simulink model "DQN_ABC_Test"  (R2023b)
settings: Solver=ode23tb  StartTime=0.0  StopTime=0.1  FixedStep=Ts  RelTol=1e-3
values from neighbouring files (symbols this model uses):
  Carm = 3.76    [DQn_ABC_Test_calc.m]
  L = Ld + Lm    [DQn_ABC_Test_calc.m]
  La = 1e-3    (= 0.001)    [DQn_ABC_Test_calc.m]
  Lb = 2*La    (= 0.002)    [DQn_ABC_Test_calc.m]
  Lc = 0.5*La    (= 0.0005)    [DQn_ABC_Test_calc.m]
  N = 1    [DQn_ABC_Test_calc.m]
  R = Rd + Rm    [DQn_ABC_Test_calc.m]
  Ra = 1.64    [DQn_ABC_Test_calc.m]
  Rb = 1.4*Ra    (= 2.296)    [DQn_ABC_Test_calc.m]
  Rc = 2.8*Ra    (= 4.592)    [DQn_ABC_Test_calc.m]
  Ta_dqn = oDP.Ta_dqn    [DQn_ABC_Test_calc.m]
  Ts = 50e-6    (= 5e-05)    [DQn_ABC_Test_calc.m]
  Ts_dqn = Ts    (= 5e-05)    [DQn_ABC_Test_calc.m]
  Ts_emt = Ts    (= 5e-05)    [DQn_ABC_Test_calc.m]
  Ws = 2*pi*f    (= 314.159265359)    [DQn_ABC_Test_calc.m]
undefined symbols (not defined in the file or in its folder): DiscIntNeverNeededParam, i, Xdcpnz, Xdcpnz_c, Xpnz, Ydcpnz, Ydcpnz_c, Ypnz
libraries: DQN_Lib x81, spsCurrentMeasurementLib x9, spsControlledVoltageSourceLib x9, spsSeriesRLCBranchLib x6, spsGroundLib x6, simulink x3, spsMutualInductanceLib x1, spspowerguiLib x1
(part 1 of 6)
settings Model: Creator=rober  LastModifiedBy=rober
settings SolverCC: ZeroCrossControl=DisableAll  DecoupledContinuousIntegration=on
settings DebuggingCC: UnconnectedInputMsg=warning  UnconnectedOutputMsg=warning  UnconnectedLineMsg=warning
settings ModelReferenceCC: EnableRefExpFcnMdlSchedulingChecks=on
settings RTWCC: DLArmComputeVersion=19.05

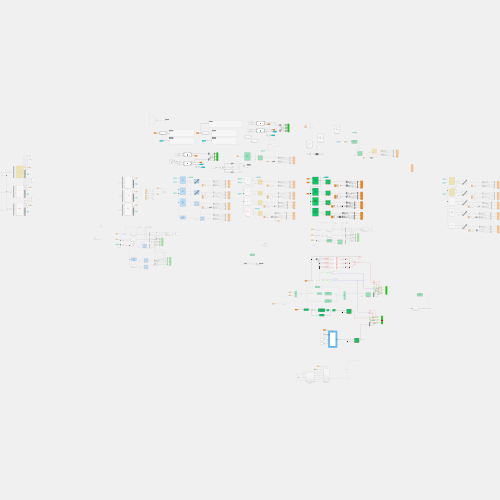
[thumbnail: Simulink's stored preview of the top-level diagram]
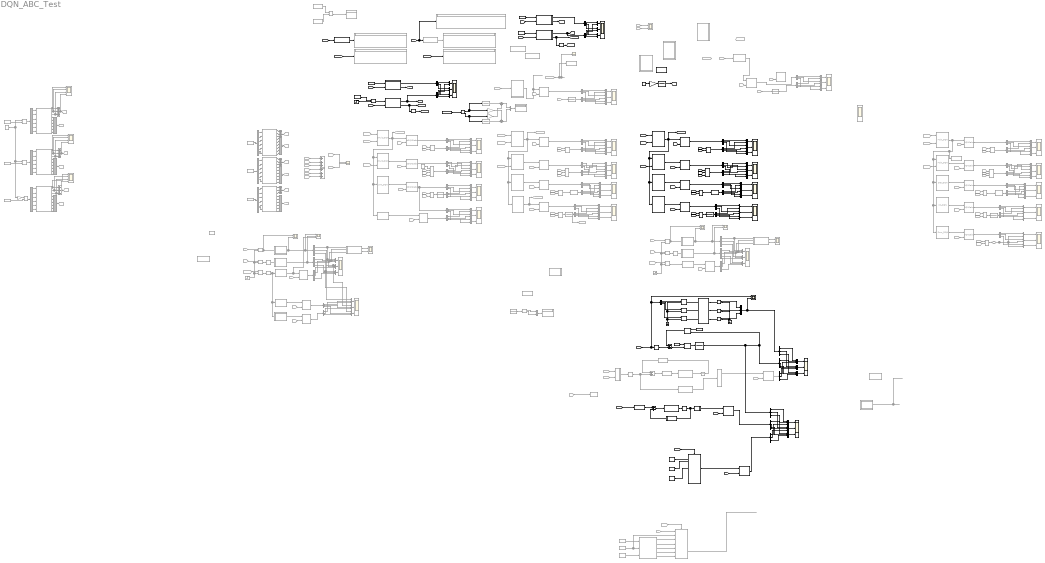
== system DQN_ABC_Test ==
  ABC : Subsystem  Commented=on
  ABC1 : Subsystem  Commented=on
  ABC2 : Subsystem  Commented=on
  Add{1..4,20..21,26..27} (8 alike) : Sum  Commented=on  Inputs=+++
  Add13 : Sum  Inputs=-+
  Add16 : Sum  Commented=on  Inputs=-+
  Add5 : Sum
  Complex to Real-Imag : ComplexToRealImag
  Complex to Real-Imag1 : ComplexToRealImag  Commented=on
  Constant : Constant  Commented=on
  Constant1 : Constant  Value=Xdcpnz
  Constant10 : Constant  Commented=on  Value=Xpnz(:,3)
  Constant11 : Constant  Value=Xdcpnz_c(1,2)
  Constant12 : Constant  Value=R
  Constant13 : Constant  Value=Xdcpnz_c
  Constant14 : Constant  Value=inv(L)
  Constant15 : Constant
  Constant16 : Constant  Value=-R/(L)
  Constant17 : Constant  Commented=on  Value=Ypnz(:,2)
  Constant18 : Constant  Commented=on  Value=Ypnz(:,3)
  Constant19 : Constant  Value=eye(3)/L
  Constant2 : Constant  Value=Ydcpnz
  Constant20 : Constant  Value=eye(3)
  Constant21 : Constant  Commented=on  Value=-R/(L)
  Constant22 : Constant  Commented=on  Value=eye(3)/L
  Constant23 : Constant  Commented=on  Value=eye(3)
  Constant3 : Constant  Commented=on
  Constant4 : Constant  Commented=on  Value=Ypnz(:,1)
  Constant5 : Constant  Value=Ydcpnz_c
  Constant6 : Constant  Commented=on  Value=Xpnz(:,1)
  Constant7 : Constant  Commented=on  Value=[1 -2 3]
  Constant8 : Constant  Commented=on  Value=[1.4 -2.8 -0.45]
  Constant9 : Constant  Commented=on  Value=Xpnz(:,2)
  Current Measurement3 : spsCurrentMeasurementLib/Current Measurement  PhasorSimulation=off  OutputType=Complex  PSBequivalent=0
  Current Measurement4 : spsCurrentMeasurementLib/Current Measurement  PhasorSimulation=off  OutputType=Complex  PSBequivalent=0
  Current Measurement5 : spsCurrentMeasurementLib/Current Measurement  PhasorSimulation=off  OutputType=Complex  PSBequivalent=0
  DQN : Subsystem  Commented=on
  DQN2abc{5,7..9} (4 alike) : DQN_Lib/DQN2abc  Commented=on  HrmOrd=2*N
  DQN2abc6 : DQN_Lib/DQN2abc  Commented=on  HrmOrd=4*N
  DQn->ABC1 : DQN_Lib/DQn->ABC19  Commented=on  N=4*N
  DQn->ABC10 : DQN_Lib/DQn->ABC19  Commented=on  N=N
  DQn->ABC{4,9,11,13} (4 alike) : DQN_Lib/DQn->ABC6  Commented=on  N=N
  DQn->ABC12 : DQN_Lib/DQn->ABC6  N=N
  DQn->ABC14 : DQN_Lib/DQn->ABC6  N=N
  DQn->ABC19 : DQN_Lib/DQn->ABC19  Commented=on  N=2*N
  DQn->ABC2 : DQN_Lib/DQn->ABC19  Commented=on  N=2*N
  DQn->ABC3 : DQN_Lib/DQn->ABC19  Commented=on  N=2*N
  DQn->ABC5 : DQN_Lib/DQn->ABC6  N=4*N
  DQn->ABC6 : DQN_Lib/DQn->ABC6  N=2*N
  DQn->ABC7 : DQN_Lib/DQn->ABC6  N=2*N
  DQn->ABC8 : DQN_Lib/DQn->ABC6  N=2*N
  Demux{,5,14..15,26..27} (6 alike) : Demux  Commented=on  Outputs=[1, 1, 1, 1, 1, 1]
  Demux{1..4,6..11,13,16..25,28..30,32..33,44..54} (37 alike) : Demux  Commented=on  Outputs=3
  Demux{12,31,34..43,55..61} (19 alike) : Demux  Outputs=3
  Demux_DQNc_Mat : DQN_Lib/Demux_DQNc_Mat  Commented=on  nrOut=2
  Der_DQN1 : DQN_Lib/Der_DQN  Commented=on  HrmOrd=2*N  FreqRad=2*pi*50  Ts=Ts_dqn  EMT=on  sw_soft=off  chkHrmLst=off  HrmLst=[7 14]
  Der_DQN_Mat : DQN_Lib/Der_DQN_Mat  Commented=on  N=2*N  w=Ws  Ts=Ts  EMT=on  sw_soft=on
  Der_DQNc_Mat : MATLAB Function  Commented=on  TreatAsAtomicUnit=on  mask{Ts=Ts, N=N, w=Ws, EMT=off, Init=zeros(3,1)}
      mask prompts: Ts "Time step (s):"; N "Harmonic order:"; w "Angular frequency [1/rad]:"; Init "Initial conditions:"
  Der_DQNc_Mat1 : DQN_Lib/Der_DQNc_Mat  Ts=Ts  N=2*N  w=Ws  EMT=on  sw_soft=on
  Discrete Derivative : simulink/Discrete/Discrete Derivative  Commented=on  gainval=1.0  ICPrevScaledInput=0.0  OutMin=[]  OutMax=[]  OutDataType=fixdt(1, 16)  OutScaling=2^-10  DoSatur=off
  Discrete Derivative1 : simulink/Discrete/Discrete Derivative  Commented=on  gainval=1.0  ICPrevScaledInput=0.0  OutMin=[]  OutMax=[]  OutDataType=fixdt(1, 16)  OutScaling=2^-10  DoSatur=off
  Discrete Derivative2 : simulink/Discrete/Discrete Derivative  gainval=1.0  ICPrevScaledInput=0.0  OutMin=[]  OutMax=[]  OutDataType=fixdt(1, 16)  OutScaling=2^-10  DoSatur=off
  Discrete-Time Integrator{,1,3,5..7,9} (7 alike) : DiscreteIntegrator  Commented=on  IntegratorMethod=Integration: Trapezoidal  SampleTime=Ts  ICPrevOutput=DiscIntNeverNeededParam  ICPrevScaledInput=DiscIntNeverNeededParam
  Discrete-Time Integrator15 : DiscreteIntegrator  IntegratorMethod=Integration: Trapezoidal  gainval=1  SampleTime=Ts_dqn  UpperSaturationLimit=5000  LowerSaturationLimit=500  ICPrevOutput=DiscIntNeverNeededParam  ICPrevScaledInput=DiscIntNeverNeededParam
  Discrete-Time Integrator2 : DiscreteIntegrator  IntegratorMethod=Integration: Trapezoidal  SampleTime=Ts  ICPrevOutput=DiscIntNeverNeededParam  ICPrevScaledInput=DiscIntNeverNeededParam
  Discrete-Time Integrator4 : DiscreteIntegrator  IntegratorMethod=Integration: Trapezoidal  SampleTime=Ts  ICPrevOutput=DiscIntNeverNeededParam  ICPrevScaledInput=DiscIntNeverNeededParam
  Discrete-Time Integrator8 : DiscreteIntegrator  Commented=on  IntegratorMethod=Integration: Trapezoidal  InitialCondition=[0.8 0.6 -0.33]  SampleTime=Ts  ICPrevOutput=DiscIntNeverNeededParam  ICPrevScaledInput=DiscIntNeverNeededParam
  Discretize BE or Tustin1 : Subsystem  Commented=on
  Display{,1,4..9} (8 alike) : Display  Commented=on
      Display settings: Decimation=1000
      Display1 settings: Decimation=1000
      Display5 settings: Decimation=1000
      Display6 settings: Decimation=1000
      Display7 settings: Decimation=1000
      Display8 settings: Decimation=1000
      Display9 settings: Decimation=1000
  EMT : Subsystem  Commented=on
  EMT1 : Subsystem  Commented=on
  Error calc : Subsystem  Commented=on
  Error calc1 : Subsystem  Commented=on
  From : From  Commented=on  GotoTag=X_DQN_mat
  From1 : From  Commented=on  GotoTag=X_DQN_vec
  From{8,10..11,15,20,43..44,46,48,50,52,54..55,57..59,81} (17 alike) : From  Commented=on  GotoTag=Yabc
  From{66,73,97,99..100,102} (6 alike) : From  Commented=on  GotoTag=Xpnz_c
  From{2,7,9,14,19,21..22,37..38,42,45,47,51,53,56,60,67,69,94..95,103..104} (22 alike) : From  Commented=on  GotoTag=Xabc
  From112 : From  Commented=on  GotoTag=X_DQN_vec
  From{3,6,12..13,16..18,30,35..36,39..41,64,72,78,89..90,98,252,262} (21 alike) : From  Commented=on  GotoTag=th0  TagVisibility=global
  From23 : From  Commented=on  GotoTag=Xabc1
  From24 : From  Commented=on  GotoTag=X_DQN_vec
  From26 : From  Commented=on  GotoTag=Xabc2
  From27 : From  Commented=on  GotoTag=Xabc3
  From28 : From  Commented=on  GotoTag=Yabc1
  From31 : From  Commented=on  GotoTag=Yabc2
  From32 : From  Commented=on  GotoTag=Yabc3
  From{4..5,33..34} (4 alike) : From  Commented=on  GotoTag=Y_DQN_vec
  From61 : From  Commented=on  GotoTag=Y_DQN_mat
  From62 : From  Commented=on  GotoTag=Y_DQN_mat
  From65 : From  Commented=on  GotoTag=iX_DQN_mat
  From68 : From  Commented=on  GotoTag=X_DQN_mat
  Gain : Gain  Gain=2*pi*50
  Gain1 : Gain  Commented=on  Gain=1/Ws
  Gain2 : Gain  Commented=on  Gain=1/Ws
  Gain8 : Gain  Commented=on
  Gain_DQNc_Mat : DQN_Lib/Gain_DQNc_Mat  Commented=on  Rabc=[R zeros(3,3); zeros(3,3) R]  HRM=N  chkInv=off
  Gain_DQNc_Mat1 : DQN_Lib/Gain_DQNc_Mat  Commented=on  Rabc=[inv(L) zeros(3,3); zeros(3,3) inv(L)]  HRM=N  chkInv=off
  Gain_DQNc_Mat2 : MATLAB Function  TreatAsAtomicUnit=on  SystemSampleTime=Ts  mask{Rabc=eye(3), HRM=N, chkInv=off}
      mask prompts: Rabc "Line matrix [3x3]:"; HRM "Harmonic order:"; chkInv "Invert"
  Gain_DQNc_Mat3 : MATLAB Function  Commented=on  TreatAsAtomicUnit=on  mask{Rabc=[L zeros(3,3); zeros(3,3) L], HRM=N, chkInv=on}
      mask prompts: Rabc "Line matrix [3x3]:"; HRM "Harmonic order:"; chkInv "Invert"
  Gain_DQNc_Mat4 : MATLAB Function  TreatAsAtomicUnit=on  SystemSampleTime=Ts  mask{Rabc=-R/(L), HRM=N, chkInv=off}
      mask prompts: Rabc "Line matrix [3x3]:"; HRM "Harmonic order:"; chkInv "Invert"
  Gain_DQNc_Mat5 : MATLAB Function  TreatAsAtomicUnit=on  SystemSampleTime=Ts  mask{Rabc=eye(3)/L, HRM=N, chkInv=off}
      mask prompts: Rabc "Line matrix [3x3]:"; HRM "Harmonic order:"; chkInv "Invert"
  Goto10 : Goto  Commented=on  GotoTag=Ydqn3
  Goto14 : Goto  Commented=on  GotoTag=XY_DQN_mat
  Goto16 : Goto  Commented=on  GotoTag=dXY_DQN_mat
  Goto17 : Goto  Commented=on  GotoTag=IntXYabc
  Goto18 : Goto  Commented=on  GotoTag=iX_DQN_mat
  Goto19 : Goto  Commented=on  GotoTag=Xabc2
  Goto2 : Goto  Commented=on  GotoTag=XY_DQN_vec
  Goto28 : Goto  Commented=on  GotoTag=Yabc2
  Goto3 : Goto  Commented=on  GotoTag=Xdqn1
  Goto32 : Goto  Commented=on  GotoTag=Xabc3
  Goto33 : Goto  Commented=on  GotoTag=Yabc3
  Goto34 : Goto  Commented=on  GotoTag=Xabc1
  Goto4 : Goto  Commented=on  GotoTag=Xdqn2
  Goto5 : Goto  Commented=on  GotoTag=Xdqn3
  Goto7 : Goto  Commented=on  GotoTag=Ydqn1
  Goto8 : Goto  Commented=on  GotoTag=Yabc1
  Goto9 : Goto  Commented=on  GotoTag=Ydqn2
  Ground2 : spsGroundLib/Ground  LConnTagsString=a
  Ground3 : spsGroundLib/Ground  LConnTagsString=a
  Ihistory_Flux : Subsystem  mask{A=-R/L, B=eye(3)/L, C=eye(3), D=zeros(3,3), Ws=2*pi*50, Ts=50e-6}
      mask prompts: Ws "Angular frequency (rad/s):"; Ts "Time step (s):"
      mask init:
      | I = eye(size(A,1));
      |     INVR = I/(I-A*Ts/2);
      |     Ad1 = INVR*(I+A*Ts/2);
      |     Bd1 = INVR*B;
      |     Cd1 = C*INVR*Ts;
      |     Dd1 = Cd1*B/2;
      | 
      |     a  = -0.5 + 1i*sqrt(3)/2;
      |     a2 = -0.5 - 1i*sqrt(3)/2;
      |     Sas = [1,a,a2;1,a2,a;1,1,1]/3;
      | 
      |     Ac = Sas*A/Sas;
      |     Bc = Sas*B/Sas;
      |     Cc = Sas*C/Sas;
      | 
      |     Ac = diag(diag(real(Ac)));
      |     Bc = diag(diag(real(Bc)));
      |     Cc = diag(diag(real(Cc)));
      settings: PortSchema="{\"entries\":[{\"content\":{\"sides\":[{\"content\":{},\"type\":\"ConnectorPlacement.EquallySpacedRectSide\",\"uuid\":\"e88392ce-eae4-4263-a591-d3f621c138f8\"},{\"content\":{\"connectorIds\":[\"Out1\"],\"side\":\"RIGHT\"},\"type\":\"ConnectorPlacement.EquallySpacedRectSide\",\"uuid\":\"cf9a43c2-5915-48ea-a98e-97bd8467efe9\"},{\"content\":{\"connectorIds\":[\"In1\"],\"side\":\"TOP\"},\"type\":\"ConnectorPlacement.EquallySpacedRectSide\",\"uuid\":\"6e30664c-e4b1-4c2e-802d-ada5c87750e1\"}]},\"type\":\"ConnectorPlacement.EquallySpacedConnector\",\"uuid\":\"d551c040-d9c0-4e4e-a3d2-ba73f5d429f0\"}],\"packageUris\":[\"http://schema.mathworks.com/mf0/Connector/R2020b\"],\"version\":\"1.0\"}"
  Ihistory_Flux1 : Subsystem  Commented=on
      settings: PortSchema="{\"entries\":[{\"content\":{\"sides\":[{\"content\":{\"connectorIds\":[\"In1\",\"In2\",\"In3\",\"In4\",\"In5\",\"In6\",\"In7\"]},\"type\":\"ConnectorPlacement.EquallySpacedRectSide\",\"uuid\":\"e88392ce-eae4-4263-a591-d3f621c138f8\"},{\"content\":{\"connectorIds\":[\"Out1\",\"Out2\"],\"side\":\"RIGHT\"},\"type\":\"ConnectorPlacement.EquallySpacedRectSide\",\"uuid\":\"cf9a43c2-5915-48ea-a98e-97bd8467efe9\"},{\"content\":{\"connectorIds\":[\"In8\"],\"side\":\"TOP\"},\"type\":\"ConnectorPlacement.EquallySpacedRectSide\",\"uuid\":\"6e30664c-e4b1-4c2e-802d-ada5c87750e1\"}]},\"type\":\"ConnectorPlacement.EquallySpacedConnector\",\"uuid\":\"d551c040-d9c0-4e4e-a3d2-ba73f5d429f0\"}],\"packageUris\":[\"http://schema.mathworks.com/mf0/Connector/R2020b\"],\"version\":\"1.0\"}"
  Int_DQN1 : DQN_Lib/Int_DQN  Commented=on  HrmOrd=2*N  FreqRad=2*pi*50  TimeStep=Ts_dqn  Init=0*(Ta_dqn*[0.01; -0.02; 0.03])'  EMT=on  chkHrmLst=off  HrmLst=[0 7 14]
  Int_DQN_Mat : DQN_Lib/Int_DQN_Mat  Commented=on  N=2*N  dt=Ts  w=Ws  EMT=off  InitInt=zeros(1,6)
  Int_DQN_Mat2 : MATLAB Function  Commented=on  TreatAsAtomicUnit=on  mask{N=N, dt=Ts, w=Ws, EMT=on, InitInt=zeros(1,6)}
      mask prompts: N "Order number:"; dt "Time step (s):"; w "Angular frequency (1/rad):"; InitInt "Initial conditions [1x6]:"
  Int_DQN_Mat4 : MATLAB Function  Commented=on  TreatAsAtomicUnit=on  mask{N=N, dt=Ts, w=Ws, EMT=on, InitInt=[0.8; 0.6; -0.33]}
      mask prompts: N "Order number:"; dt "Time step (s):"; w "Angular frequency (1/rad):"; InitInt "Initial conditions DC [3x1]:"
  Int_DQN_fdbk : DQN_Lib/Int_DQN_fdbk  Commented=on  HrmOrd=N  FreqRad=Ws  TimeStep=Ts_dqn  swFeed=on  R=Ra  iL=1/La
  Int_DQN_fdbk2 : Subsystem  Commented=on  mask{HrmOrd=N, FreqRad=Ws, TimeStep=Ts_dqn, swFeed=on, R=Ra, iL=1/La}
      mask prompts: HrmOrd "Harmonic order:"; FreqRad "Angular frequency (rad/s);"; TimeStep "Time step (s):"; swFeed "Enable feedback"; R "Feedback parameter (Kr):"; iL "Integrator parameter (Kl):"
      mask Callback swFeed:
      | EMT = get_param(gcb,'swFeed');
      | 
      | if(strcmp(EMT,'on'))
      |    set_param(gcb,'MaskVisibilities',{'on','on','on','on','on','on'});
      | else
      |    set_param(gcb,'MaskVisibilities',{'on','on','on','on','off','off'});
      | end
      mask Display:
      | %plot([0 1])
      | port_label('input',1,'{X}');
      | port_label('output',1,'{Z}');
      | 
      | harm = get_param(gcb, 'HrmOrd');
      | disp(['{\color{black}\bf\fontsize{12}Hi:',(harm),'}',newline,'{\color{red}\bf\fontsize{12}\{Int-fdbk\}}',newline,'{\color{black}\bf\fontsize{12}Ho:',(harm),'}',newline,'{\color{gray}\bf\fontsize{12}EMT}'], 'texmode','on');
  Int_DQNc_Mat : DQN_Lib/Int_DQNc_Mat  Commented=on  N=N  dt=Ts_dqn  w=Ws  InitInt=0*[0.8; 0.6; -0.33]  swFeed=on  R=diag([Ra,Rb,Rc])  iL=diag([inv(La),inv(La),inv(La)])
  Int_DQNc_Mat1 : DQN_Lib/Int_DQNc_Mat  N=2*N  dt=Ts  w=Ws  InitInt=0*[0.8; 0.6; -0.33]  swFeed=off  R=1  iL=1
  Int_DQNc_Mat2 : MATLAB Function  Commented=on  TreatAsAtomicUnit=on  mask{N=N, dt=Ts, w=Ws, InitInt=[0.8; 0.6; -0.33], swFeed=off, Ra=1, iL=1}
      mask prompts: N "Order number:"; dt "Time step (s):"; w "Angular frequency (1/rad):"; InitInt "Initial conditions DC [3x1]:"; swFeed "Enable feedback"; Ra "Feedback parameter (Kr):"; iL "Feedback parameter (Ki):"
  Int_DQNc_Mat3 : DQN_Lib/Int_DQNc_Mat  Commented=on  N=N  dt=Ts_dqn  w=Ws  InitInt=0*[0.8; 0.6; -0.33]  swFeed=off  R=Ra  iL=1/La
  Int_DQNc_Mat4 : MATLAB Function  TreatAsAtomicUnit=on  mask{N=N, dt=Ts_dqn, w=Ws, InitInt=zeros(3,1), swFeed=off, R=R/(L), iL=eye(size(-R/(L),1))}
      mask prompts: N "Order number:"; dt "Time step (s):"; w "Angular frequency (1/rad):"; InitInt "Initial conditions DC [3x1]:"; swFeed "Enable feedback"; R "Feedback parameter (Kr {abc}):"; iL "Feedback parameter (Ki {abc}):"
  Int_DQNc_Mat5 : DQN_Lib/Int_DQNc_Mat  Commented=on  N=N  dt=Ts_dqn  w=Ws  InitInt=zeros(3,1)  swFeed=on  R=[R zeros(3,3); zeros(3,3) R]  iL=[inv(L) zeros(3,3); zeros(3,3) inv(L)]
  Int_DQNc_Mat6 : DQN_Lib/Int_DQNc_Mat  Commented=on  N=N  dt=Ts_dqn  w=Ws  InitInt=zeros(3,1)  swFeed=off  R=1  iL=1
  MATLAB Function1 : MATLAB Function  TreatAsAtomicUnit=on  mask{chkHrmLst=off, HRM=N, HrmLst=[0 7 8]}
      mask prompts: chkHrmLst "Only specific harmonics"; HRM "Harmonic order:"; HrmLst "Harmonic list:"
  MATLAB Function2 : DQN_Lib/MATLAB Function4  Commented=on  SystemSampleTime=-1  VariantActivationTime=update diagram  AllowFlexibleInterface=on  Latency=0  AutoFrameSizeCalculation=off
  MATLAB Function3 : MATLAB Function  TreatAsAtomicUnit=on  mask{chkHrmLst=off, HRM=N, HrmLst=[0 7 8]}
      mask prompts: chkHrmLst "Only specific harmonics"; HRM "Harmonic order:"; HrmLst "Harmonic list:"
  MATLAB Function4 : MATLAB Function  TreatAsAtomicUnit=on  mask{chkHrmLst=off, HRM=N, HrmLst=[0 7 8]}
      mask prompts: chkHrmLst "Only specific harmonics"; HRM "Harmonic order:"; HrmLst "Harmonic list:"
  MATLAB Function6 : DQN_Lib/MATLAB Function4  SystemSampleTime=-1  VariantActivationTime=update diagram  AllowFlexibleInterface=on  Latency=0  AutoFrameSizeCalculation=off
  MATLAB Function7 : DQN_Lib/MATLAB Function4  Commented=on  SystemSampleTime=-1  VariantActivationTime=update diagram  AllowFlexibleInterface=on  Latency=0  AutoFrameSizeCalculation=off
  MATLAB Function8 : MATLAB Function  TreatAsAtomicUnit=on  mask{chkHrmLst=off, HRM=N, HrmLst=[0 7 8]}
      mask prompts: chkHrmLst "Only specific harmonics"; HRM "Harmonic order:"; HrmLst "Harmonic list:"
  MATLAB Function9 : DQN_Lib/MATLAB Function4  Commented=on  SystemSampleTime=-1  VariantActivationTime=update diagram  AllowFlexibleInterface=on  Latency=0  AutoFrameSizeCalculation=off
  Matrix Multiply8 : Product  Multiplication=Matrix(*)
  Matrix Multiply9 : Product  Multiplication=Matrix(*)
  Mult_DQN2 : DQN_Lib/Mult_DQN  Commented=on  HrmOrd=N  HrmDbl=on  chkHrmLst=off  HrmLstX=[0 7 8]  HrmLstY=[0 7 8]
  Mult_DQN3 : DQN_Lib/Mult_DQN  Commented=on  HrmOrd=2*N  HrmDbl=on  chkHrmLst=off  HrmLstX=[0 7 8 14 15 16]  HrmLstY=[0 7 8]
  Mult_DQN_Mat : DQN_Lib/Mult_DQN_Mat  Commented=on  N=N  HrmDbl=on
  Mult_DQN_Mat1 : DQN_Lib/Mult_DQN_Mat  Commented=on  N=2*N  HrmDbl=on
  Mult_DQN_Mat4 : MATLAB Function  Commented=on  TreatAsAtomicUnit=on  mask{N=N, HrmDbl=on}
      mask prompts: N "Harmonic order:"; HrmDbl "Double Harmonic"
  Mult_DQNc_Mat1 : DQN_Lib/Mult_DQNc_Mat  N=N  HrmDbl=on
  Mult_DQNc_Mat2 : DQN_Lib/Mult_DQNc_Mat  N=2*N  HrmDbl=on
  Mutual Inductance1 : spsMutualInductanceLib/Mutual Inductance  LConnTagsString=a|b|c  RConnTagsString=A|B|C  TypeOfMutual=Generalized mutual inductance  NumberOfWindings=3  SelfImpedance1=[1.1 1.1e-03]  SelfImpedance2=[ 1.1 1.1e-03]  ThreeWindings=on  SelfImpedance3=[ 1.1 1.1e-03]  MutualImpedance=[1.0 1.0e-03]  InductanceMatrix=L  ResistanceMatrix=R  Measurements=None
  Mux{,1..6,8..10,13..14,18..21,23..25,28..29,31,33..35,37..40,44..51,53..56,71..76} (47 alike) : Mux  Commented=on  Inputs=2
  Mux{7,11..12,52,57..70} (18 alike) : Mux  Inputs=2
  Mux{15..17,22,26,30} (6 alike) : Mux  Commented=on  Inputs=[1, 1, 1, 1, 1, 1]
  Mux{27,32,36,41..43,77..79} (9 alike) : Mux  Commented=on  Inputs=3
  Mux{80..86} (7 alike) : Mux  Inputs=3
  Mux_DQNc_Mat : Subsystem  Commented=on  mask{nrInp=2}
      mask prompts: nrInp "Number of inputs [{C}]"
      mask init:
      | %blocks = find_system(gcb,'LookUnderMasks','on','FollowLinks','on')
      | %set_param(gcb, 'MaskSelfModifiable', 'on');
      | 
      | % if(SSM == [])
      | %     Simulink.SubSystem.deleteContents(gcb);
      | % else
      | 
      | if(isempty(nrInp))
      |     Simulink.SubSystem.deleteContents(gcb);
      | else
      | 
      |     nrOut = 1;
      | 
      | 
      | PortHandles = get_param(gcb,'PortHandles');
      | lenInp = length(PortHandles.Inport);
      | lenOut = length(PortHandles.Inport);
      | 
      | if(nrInp ~= lenInp)
      |     %disp('ENTERED')
      |     Simulink.SubSystem.deleteContents(gcb);
      | %     add_block('simulink/Continuous/State-Space', [gcb,'/ss_block'], 'A','SS.A', 'B','SS.B', 'C','SS.C', 'D','SS.D', 'X0','X0')
      | %     set_param([gcb,'/ss_block'],'position' , [350,100,450,150])
      | 
      | 
      | 
      |         add_block('simulink/Math Operations/Matrix Concatenate',[gcb,'/Mux'], 'NumInputs',num2str(nrInp), 'ConcatenateDimension',num2str(1));
      |         set_param([gcb,'/Mux'],'position' , [200,100,250,100+nrInp*50])
      |         
      | %         add_block('built-in/Demux',[gcb,'/Demux'], 'Outputs',num2str(nrOut));
      | %         set_param([gcb,'/Demux'],'position' , [500,100,550,100+nrOut*50])
      | 
      | 
      |         for i = 1 : nrInp
      |             add_block('built-in/Inport',[gcb,strcat('/In',num2str(i))]);
      |             set_param([gcb,strcat('/In',num2str(i))],'position' , [50,65+i*50,90,85+i*50]);
      |             add_line(gcb,strcat('In',num2str(i),'/1'),strcat('Mux/',num2str(i)),'autorouting','on');
      |         end
      | 
      |         for i = 1 : nrOut
      |             add_block('built-in/Outport',[gcb,strcat('/Out',num2str(i))]);
      |             set_param([gcb,strcat('/Out',num2str(i))],'position' , [750,65+i*50,790,85+i*50]);
      |             add_line(gcb,strcat('Mux/',num2str(i)), strcat('Out',num2str(i),'/1'),'autorouting','on');
      |         end
      | 
      | 
      | %     add_line(gcb, 'Mux/1', 'ss_block/1')
      | %     add_line(gcb, 'ss_block/1', 'Demux/1')
      | 
      | end
      | 
      | end
      mask Display: disp(['{\color{red}\bf\fontsize{12}} [\{X_C\}]',newline,' MUX'], 'texmode','on');
  Product{,1,3,6..9,11..20,25,27} (19 alike) : Product  Commented=on
  Product10 : Product  Commented=on  Inputs=3
  Product2 : Product  Commented=on  Inputs=4
  Product{5,21,23..24} (4 alike) : Product
  Product22 : Product  Inputs=3
  Product4 : Product  Commented=on  Inputs=3
  Reshape : Reshape  OutputDimensionality=Customize  OutputDimensions=[N+1,6]
  Reshape1 : Reshape  OutputDimensionality=Customize  OutputDimensions=[N+1,6]
  SS_DelayPrediction : DQN_Lib/SS_DelayPrediction  N=N  Ts=Ts  x0=zeros(3,1)
  Scope{,2..3,7,13,16} (6 alike) : Scope  Commented=on  NumInputPorts=2
  Scope1 : Scope  Commented=on  NumInputPorts=4
  Scope{10..11,18,25} (4 alike) : Scope  NumInputPorts=3
  Scope12 : Scope  Commented=on
  Scope{4..6,14..15} (5 alike) : Scope  Commented=on  NumInputPorts=3
  Scope19 : Scope  NumInputPorts=2
  Scope8 : Scope  Commented=on  NumInputPorts=4
  Scope9 : Scope  Commented=on  NumInputPorts=4
  State-Space : StateSpace  Commented=on  A=-R/(L)  B=eye(3)/L  C=eye(3)  D=zeros(3,3)  InitialCondition=Ts
  Step : Step  Time=0.05  Before=1  SampleTime=0
  Step1 : Step  Commented=on  Time=0.05  Before=1  After=2  SampleTime=0
  Step2 : Step  Commented=on  Time=0.05  Before=1  After=2  SampleTime=0
  Subsystem : Subsystem  Commented=on
  Sum : Sum  Commented=on  Inputs=|++
  Sum1 : Sum  Commented=on  Inputs=+
  Sum2 : Sum  Commented=on  Inputs=-+|
  Sum_DQN1 : DQN_Lib/Sum_DQN  Commented=on  HrmOrd=2*N
  SymComp2abc_ver1 : DQN_Lib/SymComp2abc_ver2  Commented=on  H=1  f=50
  SymComp2abc_ver4 : DQN_Lib/SymComp2abc_ver2  Commented=on  H=2  f=50
  SymComp2abc_ver5 : DQN_Lib/SymComp2abc_ver2  Commented=on  H=3  f=50
  SymComp2abc_ver6 : DQN_Lib/SymComp2abc_ver2  Commented=on  H=3  f=50
  Test1 : Scope  NumInputPorts=3
  Test{2..6} (5 alike) : Scope  Commented=on  NumInputPorts=3
  Test7 : Scope  NumInputPorts=3
  To Workspace : ToWorkspace  Commented=on  VariableName=XY_DQN  SampleTime=-1
      settings: MaxDataPoints=1
  To Workspace1 : ToWorkspace  Commented=on  VariableName=Z_DQN_vec1  SaveFormat=Timeseries  SampleTime=-1
  Unit Delay1 : UnitDelay  Commented=on  SampleTime=Ts_dqn  HasFrameUpgradeWarning=on
  VS_a1 : spsControlledVoltageSourceLib/Controlled Voltage Source  Initialize=on  Source_Type=AC  Amplitude=0  Phase=0  Frequency=0  Measurements=None
  VS_b1 : spsControlledVoltageSourceLib/Controlled Voltage Source  Initialize=on  Source_Type=AC  Amplitude=0  Phase=0  Frequency=0  Measurements=None
  VS_c1 : spsControlledVoltageSourceLib/Controlled Voltage Source  Initialize=on  Source_Type=AC  Amplitude=0  Phase=0  Frequency=0  Measurements=None
  XY{,1..5,7..8} (8 alike) : Scope  Commented=on  NumInputPorts=3
  XY6 : Scope  NumInputPorts=3
  XYY : Scope  Commented=on  NumInputPorts=3
  XYY1 : Scope  Commented=on  NumInputPorts=3
  XYY2 : Scope  Commented=on  NumInputPorts=3
  XYY3 : Scope  NumInputPorts=3
  Xd1 : DQN_Lib/SymComp2abc_ver2  Commented=on  H=1  f=50
  Xd2 : DQN_Lib/SymComp2abc_ver2  Commented=on  H=2  f=50
  Zero-Order Hold1 : ZeroOrderHold  Commented=on  SampleTime=Ts_dqn
  Zero-Order Hold10 : ZeroOrderHold  Commented=on  SampleTime=Ts_dqn
  Zero-Order Hold2 : ZeroOrderHold  Commented=on  SampleTime=Ts
  Zero-Order Hold3 : ZeroOrderHold  Commented=on  SampleTime=Ts_emt
  Zero-Order Hold5 : ZeroOrderHold  Commented=on  SampleTime=Ts_emt
  Zero-Order Hold7 : ZeroOrderHold  SampleTime=Ts_dqn
  powergui : spspowerguiLib/powergui  Priority=1  SimulationMode=Discrete  SampleTime=Ts  frequency=60  Iterations=50  frequencyindice=0  Pbase=100e6  ErrMax=1e-4  UnitsV=kV  UnitsW=MW  buscounter=0  FunctionMessages=off  echomessages=off  EnableUseOfTLC=off  CurrentSourceSwitches=off  DisableSnubberDevices=off  DisableRonSwitches=off  DisableVfSwitches=off  DisplayEquations=off  AutomaticDiscreteSolvers=off  SolverType=Tustin/Backward Euler (TBE)  Interpol=off  ExternalGateDelay=off  methode=off  Ts=100  x0status=blocks  SPID=on  SwTol=0  HookPort=off  NonlinearTolerance=1e-4  nMaxIteration=100  ContinueOnMaxIteration=off  RestoreLinks=warning  ResistiveCurrentMeasurement=off  Frange=[0:2:500]  Ylog=off  Xlog=on  ShowGrid=off  save=off  variable=ZData  structure=0  ZoomFFT=off  StartTime=0.0  cycles=1  DisplayStyle=1  fundamental=60  FreqAxis=off  MaxFrequency=1000  frequencyindicesteady=1  RmsSteady=1  display=off
  sDQN2abc : DQN_Lib/sDQN2abc  Commented=on  HRM=2*N
  sDQN2abc1 : DQN_Lib/sDQN2abc  Commented=on  HRM=4*N
  sDQN2abc2 : DQN_Lib/sDQN2abc  Commented=on  HRM=2*N
  sDQN2abc4 : DQN_Lib/sDQN2abc  Commented=on  HRM=N
  sDQN2abc5 : DQN_Lib/sDQN2abc  Commented=on  HRM=N
  sDQN2abc6 : DQN_Lib/sDQN2abc  Commented=on  HRM=2*N
  sDQN2abc7 : DQN_Lib/sDQN2abc  Commented=on  HRM=N
  sInt_DQN : DQN_Lib/sInt_DQN  Commented=on  HRM=2*N  Ws=Ws  Ts=Ts  HrmSeq=off
  sInt_DQN_fdbk : DQN_Lib/sInt_DQN_fdbk  Commented=on  HRM=N  Ws=Ws  Ts=Ts_dqn  HrmSeq=off  swFeed=on  R=Ra  iL=1/La
  sInt_DQN_fdbk1 : DQN_Lib/sInt_DQN_fdbk  Commented=on  HRM=2*N  Ws=Ws  Ts=Ts  HrmSeq=off  swFeed=off  R=1  iL=1
  sMult_DQN : DQN_Lib/sMult_DQN  Commented=on  HRM=N  HrmDbl=on  HrmSeq=off
  sMult_DQN1 : DQN_Lib/sMult_DQN  Commented=on  HRM=2*N  HrmDbl=on  HrmSeq=off
  tag scope: th0=global
  wires:
  Product5/1 -> MATLAB Function3/1(Xpnz)
  Step/1 -> Product5/2
  Constant1/1 -> Product5/1
  [th0] -> MATLAB Function4/2(th)
  Constant2/1 -> MATLAB Function4/1(Xpnz)
  [th0] -> MATLAB Function3/2(th)
  Constant15/1 -> Gain/1
  Gain/1 -> Discrete-Time Integrator2/1
  Discrete-Time Integrator2/1 -> [th0]
  Mux73/1 -> XYY/2
  Mult_DQN_Mat1/1 -> DQn->ABC1/1
  From62/1 -> Mult_DQN_Mat1/2
  Demux48/3 -> Mux74/2
  Demux48/2 -> Mux73/2
  From252/1 -> DQn->ABC19/2
  Demux47/2 -> Mux54/1  "Product_b_proposed"
  Demux46/2 -> Mux54/2  "Product_b_ref"
  Demux46/3 -> Mux55/2  "Product_c_ref"
  From57/1 -> Product4/2
  Demux49/3 -> Mux74/1
  Mux56/1 -> XYY/1
  From51/1 -> Product/1
  Product4/1 -> Demux48/1  "prod"
  From58/1 -> Product4/3
  From56/1 -> Product4/1
  DQn->ABC1/1 -> Demux49/1
  From262/1 -> DQn->ABC1/2
  Demux49/2 -> Mux73/1
  Demux47/3 -> Mux55/1  "Product_c_proposed"
  Demux49/1 -> Mux56/1
  Demux48/1 -> Mux56/2
  Demux46/1 -> Mux53/2  "Product_a_ref"
  Mux53/1 -> XY/1
  Product/1 -> Demux46/1  "prod"
  From55/1 -> Product/2
  Mux74/1 -> XYY/3
  Mux54/1 -> XY/2
  Demux47/1 -> Mux53/1  "Product_a_proposed"
  Mux55/1 -> XY/3
  DQn->ABC19/1 -> Demux47/1
  Demux3/3 -> Mux6/2
  From11/1 -> Product2/4
  sDQN2abc/1 -> Demux2/1
  Mux3/1 -> XY1/3
  From4/1 -> sMult_DQN/2
  From8/1 -> Product1/2
  Demux2/1 -> Mux1/1  "Product_a_proposed"
  Demux1/1 -> Mux1/2  "Product_a_ref"
  Demux4/2 -> Mux5/1
  Mux6/1 -> XYY1/3
  Demux4/1 -> Mux4/1
  Product1/1 -> Demux1/1  "prod"
  sDQN2abc1/1 -> Demux4/1
  Mux5/1 -> XYY1/2
  Demux3/1 -> Mux4/2
  From3/1 -> sDQN2abc/2
  From7/1 -> Product1/1
  Demux1/3 -> Mux3/2  "Product_c_ref"
  Demux1/2 -> Mux2/2  "Product_b_ref"
  Mux4/1 -> XYY1/1
  Demux4/3 -> Mux6/1
  From1/1 -> sMult_DQN/1
  From5/1 -> sMult_DQN1/2
  From10/1 -> Product2/3
  Demux2/2 -> Mux2/1  "Product_b_proposed"
  Mux1/1 -> XY1/1
  Demux3/2 -> Mux5/2
  Mux2/1 -> XY1/2
  From6/1 -> sDQN2abc1/2
  Product2/1 -> Demux3/1  "prod"
  Demux2/3 -> Mux3/1  "Product_c_proposed"
  Demux45/1 -> Mux48/1  "Product_a_proposed"
  Demux45/3 -> Mux50/1  "Product_c_proposed"
  DQn->ABC3/1 -> Demux45/1
  Discrete-Time Integrator/1 -> Goto17/1, Demux44/1
  Discrete Derivative/1 -> Demux6/1
  From12/1 -> DQn->ABC3/2
  From59/1 -> Product6/2
  Mux8/1 -> Test3/1
  Mux49/1 -> Test6/2
  From81/1 -> Product7/2
  Demux44/1 -> Mux48/2  "Product_a_ref"
  Product7/1 -> Discrete-Time Integrator/1  "prod"
  Demux44/3 -> Mux50/2  "Product_c_ref"
  Product6/1 -> Discrete Derivative/1  "prod"
  Demux6/3 -> Mux10/2  "Product_c_ref"
  From60/1 -> Product7/1
  From13/1 -> DQn->ABC2/2
  Demux7/3 -> Mux10/1  "Product_c_proposed"
  From2/1 -> Product6/1
  Mux9/1 -> Test3/2
  Demux6/2 -> Mux9/2  "Product_b_ref"
  Demux7/1 -> Mux8/1  "Product_a_ref"
  Demux6/1 -> Mux8/2  "Product_a_ref"
  Demux7/2 -> Mux9/1  "Product_b_proposed"
  Mux10/1 -> Test3/3
  Mux48/1 -> Test6/1
  Demux44/2 -> Mux49/2  "Product_b_ref"
  Mux50/1 -> Test6/3
  Demux45/2 -> Mux49/1  "Product_b_proposed"
  DQn->ABC2/1 -> Demux7/1
  MATLAB Function3/2(X_DQN) -> Reshape/1, [X_DQN_vec]
  MATLAB Function4/2(X_DQN) -> [Y_DQN_vec], Reshape1/1
  From16/1 -> sDQN2abc2/2
  Product3/1 -> Discrete-Time Integrator1/1  "prod"
  Discrete-Time Integrator1/1 -> Demux10/1
  sDQN2abc2/1 -> Demux25/1, Demux11/1
  Mux21/1 -> XY3/3
  Mux19/1 -> XY3/1
  Mux20/1 -> XY3/2
  Demux11/2 -> Mux20/1  "Product_b_proposed"
  Demux11/3 -> Mux21/1  "Product_c_proposed"
  Demux10/2 -> Mux20/2  "Product_b_ref"
  Demux10/3 -> Mux21/2  "Product_c_ref"
  Demux10/1 -> Mux19/2  "Product_a_ref"
  Demux11/1 -> Mux19/1  "Product_a_proposed"
  sInt_DQN/1 -> sDQN2abc2/1
  From15/1 -> Product3/2
  From14/1 -> Product3/1
  From61/1 -> Mult_DQN_Mat/2
  From/1 -> Mult_DQN_Mat/1
  sMult_DQN/1 -> Goto2/1, sDQN2abc/1, sInt_DQN_fdbk1/1, sInt_DQN/1, sMult_DQN1/1
  From9/1 -> Product2/2
  sMult_DQN1/1 -> sDQN2abc1/1
  Constant/1 -> Product2/1
  Mult_DQN_Mat/1 -> Mult_DQN_Mat1/1, Der_DQN_Mat/1, Int_DQN_Mat/1, Goto14/1, DQn->ABC19/1
  Demux15/4 -> SymComp2abc_ver6/4
  SymComp2abc_ver5/9 -> Mux22/6
  SymComp2abc_ver1/1 -> Add2/1
  SymComp2abc_ver5/7 -> Mux22/4
  Demux15/1 -> SymComp2abc_ver6/1
  Xd1/3 -> Scope1/3, Add1/3
  Xd2/3 -> Scope8/3, Add20/3
  Product14/1 -> Demux15/1
  Demux26/5 -> SymComp2abc_ver4/5
  Add20/1 -> Scope8/4, Goto19/1
  Xd2/7 -> Mux30/4
  SymComp2abc_ver6/7 -> Mux16/4
  Demux14/5 -> Xd2/5
  Xd2/8 -> Mux30/5
  Demux27/3 -> SymComp2abc_ver5/3
  Demux14/6 -> Xd2/6
  SymComp2abc_ver1/6 -> Mux17/3
  Demux14/2 -> Xd2/2
  Xd1/7 -> Mux15/4
  Xd2/5 -> Mux30/2
  SymComp2abc_ver6/8 -> Mux16/5
  Mux26/1 -> Goto9/1
  SymComp2abc_ver5/8 -> Mux22/5
  SymComp2abc_ver5/6 -> Mux22/3
  SymComp2abc_ver4/9 -> Mux26/6
  SymComp2abc_ver5/4 -> Mux22/1
  SymComp2abc_ver5/5 -> Mux22/2
  SymComp2abc_ver4/7 -> Mux26/4
  Mux17/1 -> Goto7/1
  SymComp2abc_ver4/6 -> Mux26/3
  SymComp2abc_ver1/4 -> Mux17/1
  Xd2/6 -> Mux30/3
  Demux5/1 -> SymComp2abc_ver1/1
  Xd1/6 -> Mux15/3
  SymComp2abc_ver4/5 -> Mux26/2
  Demux15/5 -> SymComp2abc_ver6/5
  Demux/1 -> Xd1/1
  Demux/2 -> Xd1/2
  SymComp2abc_ver6/1 -> Scope9/1, Add21/1
  SymComp2abc_ver4/8 -> Mux26/5
  SymComp2abc_ver1/2 -> Add2/2
  Add27/1 -> Goto33/1
  Add26/1 -> Goto28/1
  Constant18/1 -> Demux27/1
  Demux27/1 -> SymComp2abc_ver5/1
  Xd2/1 -> Scope8/1, Add20/1
  Demux5/5 -> SymComp2abc_ver1/5
  Demux5/6 -> SymComp2abc_ver1/6
  Demux5/4 -> SymComp2abc_ver1/4
  Add1/1 -> Scope1/4, Goto34/1
  Demux14/1 -> Xd2/1
  SymComp2abc_ver5/2 -> Add27/2
  Demux27/5 -> SymComp2abc_ver5/5
  Demux27/6 -> SymComp2abc_ver5/6
  Demux15/6 -> SymComp2abc_ver6/6
  SymComp2abc_ver4/1 -> Add26/1
  Demux14/4 -> Xd2/4
  Xd1/1 -> Scope1/1, Add1/1
  SymComp2abc_ver4/2 -> Add26/2
  Demux26/1 -> SymComp2abc_ver4/1
  Demux26/3 -> SymComp2abc_ver4/3
  Constant4/1 -> Demux5/1
  Demux26/2 -> SymComp2abc_ver4/2
  Demux/3 -> Xd1/3
  SymComp2abc_ver6/5 -> Mux16/2
  Xd2/4 -> Mux30/1
  SymComp2abc_ver5/3 -> Add27/3
  Constant6/1 -> Product12/2
  Demux5/2 -> SymComp2abc_ver1/2
  SymComp2abc_ver1/9 -> Mux17/6
  Demux27/4 -> SymComp2abc_ver5/4
  Xd2/9 -> Mux30/6
  SymComp2abc_ver1/3 -> Add2/3
  Constant9/1 -> Product13/2
  Product12/1 -> Demux/1
  Constant17/1 -> Demux26/1
  SymComp2abc_ver6/3 -> Scope9/3, Add21/3
  Product13/1 -> Demux14/1
  Mux30/1 -> Goto4/1
  Demux/5 -> Xd1/5
  Xd1/9 -> Mux15/6
  SymComp2abc_ver6/9 -> Mux16/6
  SymComp2abc_ver5/1 -> Add27/1
  Constant3/1 -> Product12/1, Gain8/1, Product13/1
  Mux15/1 -> Goto3/1
  Demux26/6 -> SymComp2abc_ver4/6
  SymComp2abc_ver6/6 -> Mux16/3
  Xd2/2 -> Scope8/2, Add20/2
  Mux16/1 -> Goto5/1
  SymComp2abc_ver1/8 -> Mux17/5
  Xd1/5 -> Mux15/2
  Xd1/4 -> Mux15/1
  SymComp2abc_ver1/7 -> Mux17/4
  Demux/4 -> Xd1/4
  Demux14/3 -> Xd2/3
  Constant10/1 -> Product14/2
  Demux15/2 -> SymComp2abc_ver6/2
  Mux22/1 -> Goto10/1
  Gain8/1 -> Product14/1
  Xd1/8 -> Mux15/5
  Demux5/3 -> SymComp2abc_ver1/3
  Add2/1 -> Goto8/1
  SymComp2abc_ver6/4 -> Mux16/1
  Demux/6 -> Xd1/6
  SymComp2abc_ver4/3 -> Add26/3
  Xd1/2 -> Scope1/2, Add1/2
  SymComp2abc_ver4/4 -> Mux26/1
  Demux15/3 -> SymComp2abc_ver6/3
  Demux26/4 -> SymComp2abc_ver4/4
  Demux27/2 -> SymComp2abc_ver5/2
  SymComp2abc_ver1/5 -> Mux17/2
  From19/1 -> Scope2/1
  From20/1 -> Scope2/2
  From23/1 -> Add3/1
  From26/1 -> Add3/2
  From27/1 -> Add3/3
  From28/1 -> Add4/1
  From32/1 -> Add4/3
  From31/1 -> Add4/2
  From42/1 -> Scope/1
  From40/1 -> sDQN2abc6/2
  Demux25/1 -> Mux33/1  "Product_a_proposed"
  Demux24/2 -> Mux34/2  "Product_b_ref"
  Demux24/3 -> Mux35/2  "Product_c_ref"
  Demux24/1 -> Mux33/2  "Product_a_ref"
  Mux34/1 -> XY5/2
  Demux25/2 -> Mux34/1  "Product_b_proposed"
  sDQN2abc6/1 -> Demux24/1
  Mux35/1 -> XY5/3
  Demux25/3 -> Mux35/1  "Product_c_proposed"
  Mux33/1 -> XY5/1
  sInt_DQN_fdbk1/1 -> sDQN2abc6/1
  From43/1 -> Scope/2
  SymComp2abc_ver6/2 -> Scope9/2, Add21/2
  Add21/1 -> Scope9/4, Goto32/1
  Demux23/2 -> Mux43/2  "EMT_b_xTs"
  Step1/1 -> Product11/2, Product15/2, Product16/2
  Mux32/1 -> Scope5/1
  Demux22/3 -> Mux41/3  "DQN_c_xTs"
  Demux22/1 -> Error calc/3(DQN_a_xTs), Mux42/3  "DQN_a_xTs"
  Mux43/1 -> Scope6/2
  Mux41/1 -> Scope6/3
  Demux13/1 -> Error calc/1(EMT_a_Ts), Mux32/1, Mux42/1  "EMT_a_Ts"
  Demux19/1 -> Mux32/3  "Product_a_ref"
  Demux13/3 -> Mux27/1, Mux41/1  "EMT_c_Ts"
  Demux22/2 -> Mux43/3  "DQN_b_xTs"
  Mux42/1 -> Scope6/1
  EMT/1(Out1) -> Scope7/2, Scope4/1, Demux13/1  "I"
  Demux23/1 -> Error calc/2(EMT_a_xTs), Mux42/2  "EMT_a_xTs"
  From78/1 -> sDQN2abc4/2
  Mux36/1 -> Scope5/2
  sDQN2abc7/1 -> Demux19/1
  ABC/1(Out1) -> Scope4/2, Demux23/1
  Int_DQN_fdbk/1 -> Scope4/3, sDQN2abc4/1
  sDQN2abc5/1 -> Demux20/1
  From39/1 -> sDQN2abc5/2
  Demux20/2 -> Mux36/2  "Product_b_proposed"
  From38/1 -> Product11/1  "prod"
  Demux19/2 -> Mux36/3  "Product_b_ref"
  sDQN2abc4/1 -> Demux22/1
  Demux20/1 -> Mux32/2  "Product_a_proposed"
  Zero-Order Hold1/1 -> DQN/1(Y_DQN), sInt_DQN_fdbk/1, Int_DQN_fdbk/1
  Mux27/1 -> Scope5/3
  Product11/1 -> EMT/1(prod), Scope7/1  "V"
  Demux20/3 -> Mux27/2  "Product_c_proposed"
  From37/1 -> Product15/1  "prod"
  Demux13/2 -> Mux36/1, Mux43/1  "EMT_b_Ts"
  Error calc/2(Out2) -> Scope3/2
  Zero-Order Hold3/1 -> ABC/1(prod)
  Demux19/3 -> Mux27/3  "Product_c_ref"
  DQN/1(Out1) -> sDQN2abc7/1
  Demux23/3 -> Mux41/2  "EMT_c_xTs"
  From112/1 -> Product16/1
  From41/1 -> sDQN2abc7/2
  Product15/1 -> Zero-Order Hold3/1
  Error calc/1(Out1) -> Scope3/1
  Product16/1 -> Zero-Order Hold1/1
  sInt_DQN_fdbk/1 -> sDQN2abc5/1
  Reshape1/1 -> [Y_DQN_mat]
  Demux18/3 -> Mux31/1  "Product_c_proposed"
  Demux16/2 -> Mux24/1  "Product_b_proposed"
  Demux16/1 -> Mux23/1  "Product_a_proposed"
  Mux44/1 -> Test4/1
  DQN2abc6/1 -> Demux28/1
  From46/1 -> Product8/2
  Demux16/3 -> Mux25/1  "Product_c_proposed"
  Mux13/1 -> Test4/3
  Int_DQN1/1 -> DQN2abc8/1
  DQN2abc5/1 -> Demux18/1
  Demux18/1 -> Mux28/1  "Product_a_proposed"
  Mux24/1 -> Test5/2
  Sum_DQN1/1 -> DQN2abc9/1
  Demux29/3 -> Mux13/2  "Product_c_ref"
  Mux40/1 -> XYY2/3
  Sum1/1 -> Mux18/2, Mux38/2, Mux14/2  "Product_c_ref"
  From35/1 -> DQN2abc6/2
  Mux25/1 -> Test5/3
  From34/1 -> Mult_DQN3/2
  Mux31/1 -> XY2/3
  From48/1 -> Product10/2
  Discrete-Time Integrator3/1 -> Demux9/1
  Mux37/1 -> XYY2/1
  Demux28/3 -> Mux40/1
  From17/1 -> DQN2abc8/2
  Mux14/1 -> Test2/2
  From30/1 -> DQN2abc5/2
  Discrete Derivative1/1 -> Demux29/1
  Mux45/1 -> Test4/2
  Demux18/2 -> Mux29/1  "Product_b_proposed"
  Demux17/3 -> Mux31/2  "Product_c_ref"
  From22/1 -> Product19/1
  Demux21/3 -> Mux40/2
  Demux8/3 -> Mux18/1  "Product_c_proposed"
  Demux30/1 -> Mux44/1  "Product_a_ref"
  DQN2abc7/1 -> Demux30/1
  From44/1 -> Product19/2
  Mux23/1 -> Test5/1
  Demux17/2 -> Mux29/2  "Product_b_ref"
  From36/1 -> DQN2abc9/2
  Demux8/2 -> Mux14/1  "Product_b_proposed"
  Mux38/1 -> Test2/1
  DQN2abc9/1 -> Demux8/1
  From24/1 -> Mult_DQN2/1
  Product17/1 -> Discrete Derivative1/1  "prod"
  DQN2abc8/1 -> Demux16/1
  Demux30/3 -> Mux13/1  "Product_c_proposed"
  Demux8/1 -> Mux38/1  "Product_a_proposed"
  Demux29/1 -> Mux44/2  "Product_a_ref"
  Demux9/2 -> Mux24/2  "Product_b_ref"
  Product10/1 -> Demux21/1  "prod"
  Demux29/2 -> Mux45/2  "Product_b_ref"
  Demux21/2 -> Mux39/2
  From21/1 -> Product17/1
  From54/1 -> Product18/2
  From53/1 -> Product18/1
  Demux9/3 -> Mux25/2  "Product_c_ref"
  From18/1 -> DQN2abc7/2
  From45/1 -> Product8/1
  From47/1 -> Product10/1
  Demux9/1 -> Mux23/2  "Product_a_ref"
  Demux30/2 -> Mux45/1  "Product_b_proposed"
  Der_DQN1/1 -> DQN2abc7/1
  Demux28/1 -> Mux37/1
  Product8/1 -> Demux17/1  "prod"
  Demux28/2 -> Mux39/1
  From50/1 -> Product10/3
  Demux21/1 -> Mux37/2
  Mult_DQN3/1 -> DQN2abc6/1
  Mult_DQN2/1 -> To Workspace1/1, Sum_DQN1/1, Int_DQN1/1, Der_DQN1/1, Mult_DQN3/1, DQN2abc5/1
  Demux17/1 -> Mux28/2  "Product_a_ref"
  Mux29/1 -> XY2/2
  Mux18/1 -> Test2/3
  From52/1 -> Product17/2
  Product19/1 -> Sum1/1  "prod"
  Mux28/1 -> XY2/1
  Mux39/1 -> XYY2/2
  Product18/1 -> Discrete-Time Integrator3/1  "prod"
  From33/1 -> Mult_DQN2/2
  Reshape/1 -> [X_DQN_mat]
  MATLAB Function8/2(Xpnz_c) -> [Xpnz_c]
  [th0] -> MATLAB Function8/2(tho)
  Constant13/1 -> MATLAB Function8/1(Xpnz_ci)
  Mux12/1 -> Scope10/1
  Mux11/1 -> Scope10/2
  Demux31/3 -> Mux7/1
  Demux12/3 -> Mux7/2
  Demux12/1 -> Mux12/2
  MATLAB Function3/1(Xabc) -> Demux12/1, [Xabc]
  Mux7/1 -> Scope10/3
  Demux12/2 -> Mux11/2
  Demux31/1 -> Mux12/1
  MATLAB Function8/1(Xabc) -> Demux31/1
  Demux31/2 -> Mux11/1
  [X_DQN_mat] -> Display/1
  [Xpnz_c] -> MATLAB Function6/1
  MATLAB Function6/1 -> Display1/1
  Der_DQNc_Mat/1(Zpnz) -> DQn->ABC9/1
  DQn->ABC9/1 -> Demux33/1
  Demux33/3 -> Mux51/1  "Product_c_proposed"
  Demux33/1 -> Mux46/1  "Product_a_proposed"
  Mux51/1 -> XY4/3
  Demux32/2 -> Mux47/2  "Product_b_ref"
  Demux33/2 -> Mux47/1  "Product_b_proposed"
  Demux32/3 -> Mux51/2  "Product_c_ref"
  From67/1 -> Discrete-Time Integrator9/1  "prod"
  Demux32/1 -> Mux46/2  "Product_a_ref"
  Mux47/1 -> XY4/2
  Mux46/1 -> XY4/1
  From64/1 -> DQn->ABC9/2
  [th0] -> MATLAB Function1/2(tho)
  Constant5/1 -> MATLAB Function1/1(Xpnz_ci)
  MATLAB Function1/2(Xpnz_c) -> [Ypnz_c]
  MATLAB Function1/1(Xabc) -> Demux35/1
  MATLAB Function4/1(Xabc) -> Demux34/1, [Yabc]
  Demux35/2 -> Mux52/1
  Demux34/2 -> Mux52/2
  Demux34/1 -> Mux57/2
  Demux35/1 -> Mux57/1
  Mux58/1 -> Scope11/3
  Mux52/1 -> Scope11/2
  Mux57/1 -> Scope11/1
  Demux35/3 -> Mux58/1
  Demux34/3 -> Mux58/2
  Constant7/1 -> Product20/1
  Constant8/1 -> Product20/2
  Product20/1 -> Display4/1
  From65/1 -> To Workspace/1, Scope12/1
  MATLAB Function7/1 -> Display6/1
  [Y_DQN_mat] -> Display5/1
  [Ypnz_c] -> Display9/1, MATLAB Function7/1
  Demux40/3 -> Mux68/2
  [Ypnz_c] -> Mult_DQNc_Mat2/2
  Mult_DQNc_Mat2/1 -> DQn->ABC5/1
  Mux67/1 -> XYY3/2
  DQn->ABC5/1 -> Demux41/1
  Demux39/1 -> Mux63/1  "Product_a_proposed"
  [Xabc] -> Product22/1
  Demux41/2 -> Mux67/1
  [Ypnz_c] -> Mult_DQNc_Mat1/2
  Demux41/1 -> Mux66/1
  [th0] -> DQn->ABC7/2
  [Yabc] -> Product22/3
  [Yabc] -> Product24/2
  Demux42/1 -> Mux69/2  "Product_a_ref"
  Mult_DQNc_Mat1/1 -> DQn->ABC6/1, Mult_DQNc_Mat2/1, Int_DQNc_Mat1/1, Der_DQNc_Mat1/1, [XY_DQNc_mat]
  [Xpnz_c] -> Mult_DQNc_Mat1/1
  Mux61/1 -> Test7/2
  [Yabc] -> Product23/2
  Demux42/2 -> Mux70/2  "Product_b_ref"
  [Xabc] -> Product24/1
  Demux37/1 -> Mux60/1  "Product_a_proposed"
  Discrete Derivative2/1 -> Demux42/1
  Der_DQNc_Mat1/1 -> DQn->ABC7/1
  Demux37/2 -> Mux61/1  "Product_b_proposed"
  Int_DQNc_Mat1/1 -> DQn->ABC8/1
  Discrete-Time Integrator4/1 -> Demux36/1
  Mux68/1 -> XYY3/3
  Mux64/1 -> XY6/2
  DQn->ABC6/1 -> Demux39/1
  [Xabc] -> Product23/1
  Demux38/1 -> Mux63/2  "Product_a_ref"
  Product21/1 -> Demux38/1  "prod"
  [Yabc] -> Product21/2
  [th0] -> DQn->ABC5/2
  Demux42/3 -> Mux59/2  "Product_c_ref"
  Demux36/3 -> Mux62/2  "Product_c_ref"
  [Yabc] -> Product22/2
  DQn->ABC8/1 -> Demux37/1
  DQn->ABC7/1 -> Demux43/1
  Mux63/1 -> XY6/1
  Mux70/1 -> Test1/2
  Demux40/1 -> Mux66/2
  [Xabc] -> Product21/1
  Demux38/3 -> Mux65/2  "Product_c_ref"
  Mux66/1 -> XYY3/1
  Demux38/2 -> Mux64/2  "Product_b_ref"
  Demux39/2 -> Mux64/1  "Product_b_proposed"
  Demux43/1 -> Mux69/1  "Product_a_ref"
  Mux65/1 -> XY6/3
  Mux62/1 -> Test7/3
  [th0] -> DQn->ABC8/2
  Mux60/1 -> Test7/1
  Demux43/2 -> Mux70/1  "Product_b_proposed"
  Product23/1 -> Discrete Derivative2/1  "prod"
  Demux43/3 -> Mux59/1  "Product_c_proposed"
  Product24/1 -> Discrete-Time Integrator4/1  "prod"
  Demux39/3 -> Mux65/1  "Product_c_proposed"
  Mux69/1 -> Test1/1
  Demux37/3 -> Mux62/1  "Product_c_proposed"
  Demux41/3 -> Mux68/1
  Product22/1 -> Demux40/1  "prod"
  Mux59/1 -> Test1/3
  Demux36/1 -> Mux60/2  "Product_a_ref"
  Demux36/2 -> Mux61/2  "Product_b_ref"
  Demux40/2 -> Mux67/2
  [th0] -> DQn->ABC6/2
  Der_DQN_Mat/1 -> DQn->ABC2/1
  From66/1 -> Der_DQNc_Mat/1(Xpnz)
  Int_DQN_Mat/1 -> Goto16/1, DQn->ABC3/1
  Discrete-Time Integrator7/1 -> Complex to Real-Imag1/1
  Complex to Real-Imag1/1 -> Mux71/1
  Mux71/1 -> Display8/1
  Complex to Real-Imag1/2 -> Mux71/2
  Demux50/3 -> Mux76/2  "Product_c_ref"
  Mux75/1 -> XY8/2
  Demux51/3 -> Mux76/1  "Product_c_proposed"
  Mux72/1 -> XY8/1
  Mux76/1 -> XY8/3
  Demux50/2 -> Mux75/2  "Product_b_ref"
  From69/1 -> Discrete-Time Integrator8/1
  Demux50/1 -> Mux72/2  "Product_a_ref"
  Demux51/2 -> Mux75/1  "Product_b_proposed"
  Demux51/1 -> Mux72/1  "Product_a_proposed"
  Discrete-Time Integrator8/1 -> Demux50/1
  Discrete-Time Integrator9/1 -> Demux32/1
  Mux/1 -> Display7/1
  Constant11/1 -> Complex to Real-Imag/1
  Complex to Real-Imag/1 -> Gain2/1, Discrete-Time Integrator5/1
  Sum/1 -> Mux/1
  Complex to Real-Imag/2 -> Gain1/1, Discrete-Time Integrator6/1
  Gain1/1 -> Sum/2
  Sum2/1 -> Mux/2
  Gain2/1 -> Sum2/1
  Discrete-Time Integrator6/1 -> Sum2/2
  Discrete-Time Integrator5/1 -> Sum/1
  From73/1 -> Int_DQNc_Mat2/1(Xpnz)
  From72/1 -> DQn->ABC10/2
  From89/1 -> DQn->ABC4/2
  Int_DQNc_Mat2/1(Zpnz) -> DQn->ABC4/1
  DQn->ABC4/1 -> Demux51/1
  Demux54/1 -> Error calc1/2(EMT_a_xTs), Mux78/2  "EMT_a_xTs"
  Error calc1/1(Out1) -> Scope13/1
  Mux77/1 -> Scope15/3
  Step2/1 -> Product9/2, Product25/2, Product27/2
  Demux54/2 -> Mux79/2  "EMT_b_xTs"
  Mux79/1 -> Scope15/2
  ABC1/1(Out1) -> Scope14/2, Demux54/1
  Error calc1/2(Out2) -> Scope13/2
  From95/1 -> Product9/1  "prod"
  From94/1 -> Product25/1  "prod"
  Demux54/3 -> Mux77/2  "EMT_c_xTs"
  Product25/1 -> Zero-Order Hold5/1
  Demux53/2 -> Mux79/3  "DQN_b_xTs"
  Mux78/1 -> Scope15/1
  Demux53/3 -> Mux77/3  "DQN_c_xTs"
  EMT1/1(Out1) -> Scope16/2, Scope14/1, Demux52/1  "I"
  Demux53/1 -> Error calc1/3(DQN_a_xTs), Mux78/3  "DQN_a_xTs"
  Demux52/2 -> Mux79/1  "EMT_b_Ts"
  Zero-Order Hold5/1 -> ABC1/1(prod)
  Demux52/1 -> Error calc1/1(EMT_a_Ts), Mux78/1  "EMT_a_Ts"
  Demux52/3 -> Mux77/1  "EMT_c_Ts"
  Product9/1 -> EMT1/1(prod), Scope16/1  "V"
  From98/1 -> DQn->ABC11/2
  Int_DQNc_Mat/1 -> DQn->ABC11/1
  DQn->ABC11/1 -> Demux53/1
  Product27/1 -> Int_DQNc_Mat/1
  From97/1 -> Product27/1
  Mux83/1 -> Scope25/2
  Current Measurement4/1 -> Mux80/2
  Demux58/1 -> VS_a1/1
  Gain_DQNc_Mat1/1 -> Int_DQNc_Mat6/1
  Demux57/1 -> Mux82/2  "EMT_a_xTs"
  Matrix Multiply8/1 -> Add13/1
  Zero-Order Hold7/1 -> Add13/2
  Constant14/1 -> Matrix Multiply9/1
  Demux56/3 -> Mux81/3  "DQN_c_xTs"
  Demux55/2 -> Mux83/1  "EMT_b_Ts"
  Int_DQNc_Mat6/1 -> Unit Delay1/1
  Matrix Multiply9/1 -> Discrete-Time Integrator15/1
  Demux55/3 -> Mux81/1  "EMT_c_Ts"
  Demux57/2 -> Mux83/2  "EMT_b_xTs"
  Demux55/1 -> Mux82/1  "EMT_a_Ts"
  Demux58/3 -> VS_c1/1
  Unit Delay1/1 -> Gain_DQNc_Mat/1
  Mux81/1 -> Scope25/3
  Constant12/1 -> Matrix Multiply8/1
  [Xabc] -> Zero-Order Hold7/1, Demux58/1, Scope19/1  "prod"
  Current Measurement5/1 -> Mux80/3
  Current Measurement3/1 -> Mux80/1
  Demux58/2 -> VS_b1/1
  Demux56/2 -> Mux83/3  "DQN_b_xTs"
  Add16/1 -> Gain_DQNc_Mat1/1
  Demux56/1 -> Mux82/3  "DQN_a_xTs"
  Add13/1 -> Matrix Multiply9/2
  Mux80/1 -> Demux55/1, Scope19/2
  From90/1 -> DQn->ABC13/2
  Demux57/3 -> Mux81/2  "EMT_c_xTs"
  Mux82/1 -> Scope25/1
  DQn->ABC13/1 -> Demux56/1
  From99/1 -> Mux_DQNc_Mat/1(In1)
  Mux_DQNc_Mat/1(Out1) -> Zero-Order Hold10/1
  Demux_DQNc_Mat/1 -> DQn->ABC13/1
  Gain_DQNc_Mat/1 -> Add16/1
  ABC2/1(Out1) -> ?
  ? -> ABC2/1(prod)
  From100/1 -> Mux_DQNc_Mat/2(In2)
  Int_DQNc_Mat5/1 -> Demux_DQNc_Mat/1
  Zero-Order Hold10/1 -> Int_DQNc_Mat5/1, Add16/2
  From104/1 -> State-Space/1  "prod"
  Demux61/1 -> Mux85/2  "EMT_a_xTs"
  Mux86/1 -> Scope18/2
  Demux61/2 -> Mux86/2  "EMT_b_xTs"
  Demux61/3 -> Mux84/2  "EMT_c_xTs"
  Demux60/2 -> Mux86/3  "DQN_b_xTs"
  Demux60/1 -> Mux85/3  "DQN_a_xTs"
  Mux85/1 -> Scope18/1
  Mux84/1 -> Scope18/3
  Demux59/1 -> Mux85/1  "EMT_a_Ts"
  Demux59/2 -> Mux86/1  "EMT_b_Ts"
  Demux59/3 -> Mux84/1  "EMT_c_Ts"
  Demux60/3 -> Mux84/3  "DQN_c_xTs"
  Discrete-Time Integrator15/1 -> Demux59/1, Demux57/1, Matrix Multiply8/2
  [Xpnz_c] -> Gain_DQNc_Mat5/1(Xpnz)
  Int_DQNc_Mat4/1(Zpnz) -> SS_DelayPrediction/1
  SS_DelayPrediction/1 -> Gain_DQNc_Mat2/1(Xpnz), Gain_DQNc_Mat4/1(Xpnz)  "dw"
  Add5/1 -> Int_DQNc_Mat4/1(Xpnz)
  Gain_DQNc_Mat4/1(Ypnz) -> Add5/2
  Gain_DQNc_Mat5/1(Ypnz) -> Add5/1
  Gain_DQNc_Mat2/1(Ypnz) -> DQn->ABC14/1
  [th0] -> DQn->ABC14/2
  DQn->ABC14/1 -> Demux61/1
  Constant19/1 -> ?
  Constant16/1 -> ?
  Constant20/1 -> ?
  DQn->ABC12/1 -> Demux60/1  "I(k) = Linv*phi"
  [Xpnz_c] -> Ihistory_Flux/1(u_c)
  From102/1 -> Ihistory_Flux1/8(u_c)
  Ihistory_Flux1/2(phi) -> ?  "I(k) = Linv*phi"
  Constant23/1 -> Discretize BE or Tustin1/3(C)
  Discretize BE or Tustin1/5(inv(I_Ts/2*A)) -> Ihistory_Flux1/7(inv())
  From103/1 -> Ihistory_Flux1/1(u)  "prod"
  Constant21/1 -> Discretize BE or Tustin1/1(A)
  Constant22/1 -> Ihistory_Flux1/2(B), Discretize BE or Tustin1/2(B)
  Discretize BE or Tustin1/4(Dd) -> Ihistory_Flux1/6(Dd)
  Discretize BE or Tustin1/3(Cd) -> Ihistory_Flux1/5(Cd)
  Discretize BE or Tustin1/1(Ad) -> Ihistory_Flux1/3(Ad)
  Discretize BE or Tustin1/2(Bd) -> Ihistory_Flux1/4(Bd)
  [th0] -> DQn->ABC12/2
  Ihistory_Flux/1(Yc) -> DQn->ABC12/1  "I(k) = Linv*phi"
  connections:
  VS_c1/LConn1 -- Ground2/LConn1 -- VS_a1/LConn1 -- VS_b1/LConn1
  Ground3/LConn1 -- Current Measurement4/RConn1 -- Current Measurement3/RConn1 -- Current Measurement5/RConn1
  Mutual Inductance1/LConn1 -- VS_a1/RConn1
  Mutual Inductance1/RConn2 -- Current Measurement4/LConn1
  Mutual Inductance1/LConn2 -- VS_b1/RConn1
  Mutual Inductance1/RConn3 -- Current Measurement5/LConn1
  Mutual Inductance1/LConn3 -- VS_c1/RConn1
  Mutual Inductance1/RConn1 -- Current Measurement3/LConn1

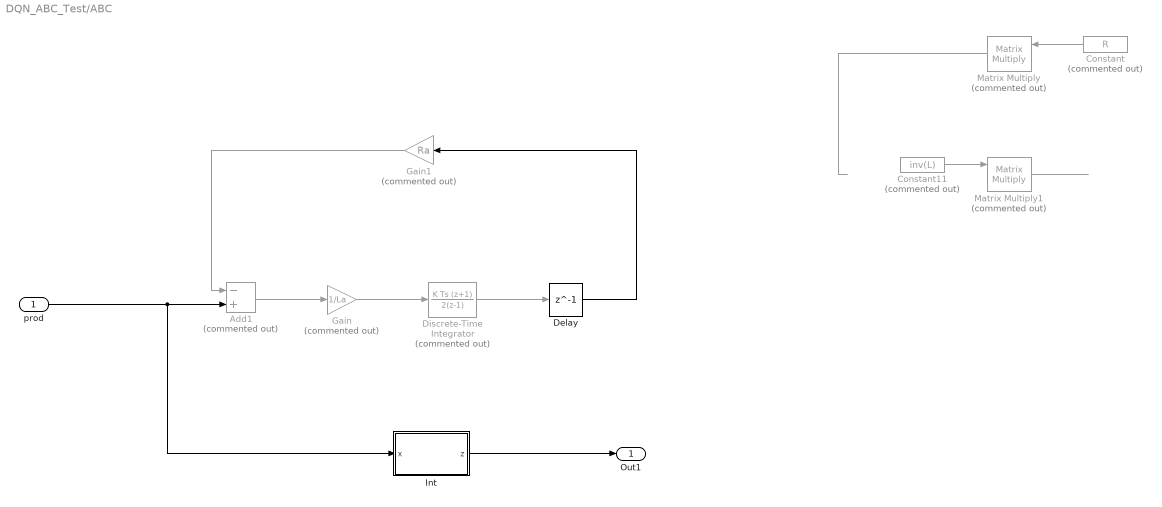
== system DQN_ABC_Test/ABC ==
  prod : Inport
  Add1 : Sum  Commented=on  Inputs=-+
  Constant : Constant  Commented=on  Value=R
  Constant11 : Constant  Commented=on  Value=inv(L)
  Delay : Delay  DelayLength=1
  Discrete-Time Integrator : DiscreteIntegrator  Commented=on  IntegratorMethod=Integration: Trapezoidal  SampleTime=Ts_emt  ICPrevOutput=DiscIntNeverNeededParam  ICPrevScaledInput=DiscIntNeverNeededParam
  Gain : Gain  Commented=on  Gain=1/La
  Gain1 : Gain  Commented=on  Gain=Ra
  Int : MATLAB Function  TreatAsAtomicUnit=on  mask{dt=Ts_emt}
      mask prompts: dt "Time step (s):"
  Matrix Multiply : Product  Commented=on  Multiplication=Matrix(*)
  Matrix Multiply1 : Product  Commented=on  Multiplication=Matrix(*)
  Out1 : Outport
  wires:
  prod/1 -> Int/1(x), Add1/2
  ? -> Matrix Multiply1/2
  Constant11/1 -> Matrix Multiply1/1
  Constant/1 -> Matrix Multiply/1
  Matrix Multiply1/1 -> ?
  Matrix Multiply/1 -> ?
  ? -> Matrix Multiply/2
  Add1/1 -> Gain/1
  Int/1(z) -> Out1/1
  Gain1/1 -> Add1/1
  Gain/1 -> Discrete-Time Integrator/1
  Discrete-Time Integrator/1 -> Delay/1
  Delay/1 -> Gain1/1
